simulink model "serial_comms_test"  (R2020a)
settings: Solver=ode4  StartTime=0.0  StopTime=100.0  FixedStep=0.001  RelTol=1e-3
undefined symbols (not defined in the file): serial
libraries: instrumentlib x3, xpcseriallib x1
settings Model: EnablePacing=on  Creator=Jared  LastModifiedBy=Mason
settings DataIOCC: ReturnWorkspaceOutputs=off
settings DebuggingCC: ArithmeticOperatorsInVariantConditions=warning
settings SFSimCC: CustomCodeUndefinedFunction=UseInterfaceOnly

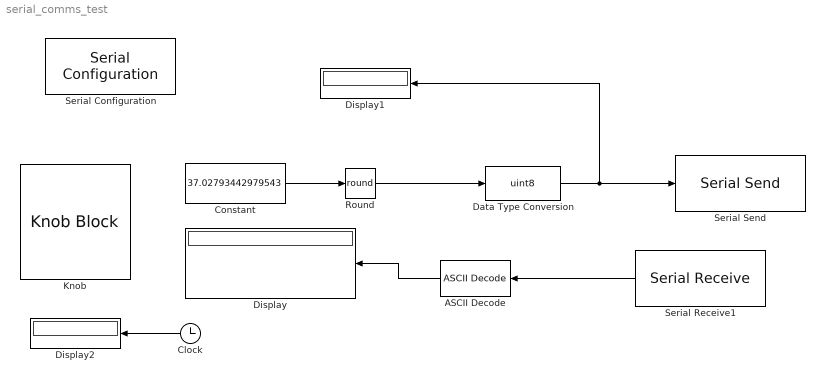
== system serial_comms_test ==
  "ASCII Decode " : xpcseriallib/ASCII Decode   format=%d\r  nvars=1  vartypes={ }
      settings: SourceProductBaseCode=XP
  Clock : Clock
  Constant : Constant  Value=37.02793442979543  OutDataTypeStr=double  SampleTime=0.5
  Data Type Conversion : DataTypeConversion  OutDataTypeStr=uint8  SaturateOnIntegerOverflow=on
  Display : Display
  Display1 : Display
  Display2 : Display
  Knob : KnobBlock  ScaleMax=50
  Round : Rounding  Operator=round
  Serial Configuration : instrumentlib/Serial Configuration  Priority=-200000  ComPortMenu=COM3  ComPort=COM3  ObjConstructor=serial('COM3');  BaudRate=9600  DataBits=8  Parity=none  StopBits=1  FlowControl=none  Timeout=10  ByteOrder=LittleEndian
  Serial Receive1 : instrumentlib/Serial Receive  ComPortMenu=COM3  ComPort=COM3  ObjConstructor=serial('COM3');  Terminator=<none>  DataSize="[2  1]"  DataType=uint8  EnableBlockingMode=on  ActionDataUnavailable=Output custom value  CustomValue=9  SampleTime=0.5
  Serial Send : instrumentlib/Serial Send  ComPortMenu=COM3  ComPort=COM3  ObjConstructor=serial('COM3');  Terminator=<none>  EnableBlockingMode=on
  wires:
  Serial Receive1/1 -> "ASCII Decode "/1
  Clock/1 -> Display2/1
  Constant/1 -> Round/1
  "ASCII Decode "/1 -> Display/1
  Round/1 -> Data Type Conversion/1
  Data Type Conversion/1 -> Display1/1, Serial Send/1
